simulink library "Power_Electronic_Lab_Controllers"  (R2019b)
settings: Solver=VariableStepAuto  StartTime=0.0  StopTime=10.0  RelTol=1e-3
settings Model: Creator=mehdi  LastModifiedBy=mehdi

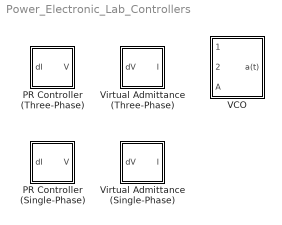
== system Power_Electronic_Lab_Controllers ==
  PR Controller (Single-Phase) : Subsystem  mask{Kp=0.1, Kr=0.2, w0=100*pi}
      mask prompts: Kp "Proportional Gain"; Kr "Resonant Gain"; w0 "Mid Angular Freqeuncy"
      mask DialogControl DescGroupVar Prompt: PR Controller
      mask DialogControl DescTextVar1 Prompt: This Type of controller used as PI Controller but for Sinosoidal input with Angular Freqeunce near by w0.
      mask DialogControl DescTextVar Prompt: The controller desined with 2 parameter Kp and Kr. To understand and desing this controller plot bode diagram from controller transfer function.
  PR Controller (Three-Phase) : Subsystem  mask{Kp=0.1, Kr=0.2, w0=100*pi}
      mask prompts: Kp "Proportional Gain"; Kr "Resonant Gain"; w0 "Mid Angular Freqeuncy"
      mask DialogControl DescGroupVar Prompt: PR Controller
      mask DialogControl DescTextVar1 Prompt: This Type of controller used as PI Controller but for Sinosoidal input with Angular Freqeunce near by w0.
      mask DialogControl DescTextVar Prompt: The controller desined with 2 parameter Kp and Kr. To understand and desing this controller plot bode diagram from controller transfer function.
  VCO : Subsystem  mask{input_sel=Freq. and Arc, pn_sel=Posetive, arc_type_sel=cos, k=-2.0944, theta0=1.5708}
      mask prompts: input_sel "Arc"; pn_sel "Sequence"; arc_type_sel "Function"
      mask TypeOptions input_sel: Arc Only | Freq. Only | Freq. and Arc
      mask Callback input_sel: VCO_Callback()
      mask TypeOptions pn_sel: Posetive | Negetive
      mask Callback pn_sel:
      | sel=get_param(gcb, 'pn_sel');
      | if strcmp(sel, 'Posetive')
      |     set_param(gcb, 'k', num2str(-2*pi/3))
      | else
      |     set_param(gcb, 'k', num2str(+2*pi/3))
      | end
      mask TypeOptions arc_type_sel: sin | cos
      mask Callback arc_type_sel:
      | type=get_param(gcb, 'arc_type_sel');
      | if strcmp(type, 'sin')
      |     set_param(gcb, 'theta0', num2str(0))
      | else
      |     set_param(gcb, 'theta0', num2str(pi/2))
      | end
      mask DialogControl Container2 Prompt: Hidden Parameters
      mask Display:
      | sel=get_param(gcb,  'input_sel');
      | 
      | switch sel
      | case 'Arc Only'
      |     port_label('input', 1, '\theta', 'texmode', 'on')
      | case 'Freq. Only'
      |     port_label('input', 1, '\omega', 'texmode', 'on')
      | case 'Freq. and Arc'
      |     port_label('input', 1, '\theta', 'texmode', 'on')
      |     port_label('input', 2, '\omega', 'texmode', 'on')
      | end
  Virtual Admittance (Single-Phase) : Subsystem  mask{R=0.05, X=0.1, Zb=1.6, w0=100*pi}
      mask prompts: R "R (pu)"; X "X (pu)"; w0 "Angelur Frequency"
      mask DialogControl DescGroupVar Prompt: Virtual Admmitance
      mask DialogControl DescTextVar Prompt: This module is one of control structures of Grig Feeder and used for calculate refrence current from actual voltage of inverter and VCO output.
  Virtual Admittance (Three-Phase) : Subsystem  mask{R=0.05, X=0.1, Zb=1.6, w0=100*pi}
      mask prompts: R "R (pu)"; X "X (pu)"; w0 "Angelur Frequency"
      mask DialogControl DescGroupVar Prompt: Virtual Admmitance
      mask DialogControl DescTextVar Prompt: This module is one of control structures of Grig Feeder and used for calculate refrence current from actual voltage of inverter and VCO output.

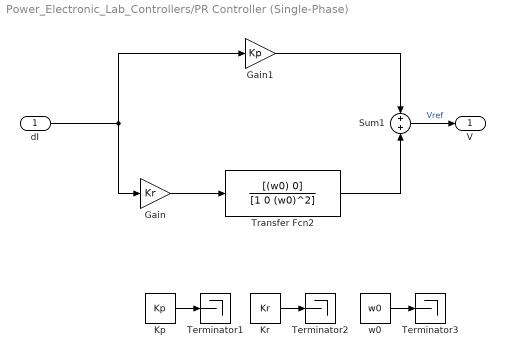
== system Power_Electronic_Lab_Controllers/PR Controller (Single-Phase) ==
  dI : Inport
  Gain : Gain  Gain=Kr
  Gain1 : Gain  Gain=Kp
  Kp : Constant  Value=Kp
  Kr : Constant  Value=Kr
  Sum1 : Sum
  Terminator1 : Terminator
  Terminator2 : Terminator
  Terminator3 : Terminator
  Transfer Fcn2 : TransferFcn  Numerator=[(w0) 0]  Denominator=[1 0 (w0)^2]
  w0 : Constant  Value=w0
  V : Outport  VectorParamsAs1DForOutWhenUnconnected=off
  wires:
  Transfer Fcn2/1 -> Sum1/2
  Gain/1 -> Transfer Fcn2/1
  Kr/1 -> Terminator2/1
  Kp/1 -> Terminator1/1
  w0/1 -> Terminator3/1
  dI/1 -> Gain1/1, Gain/1
  Gain1/1 -> Sum1/1
  Sum1/1 -> V/1  "Vref"

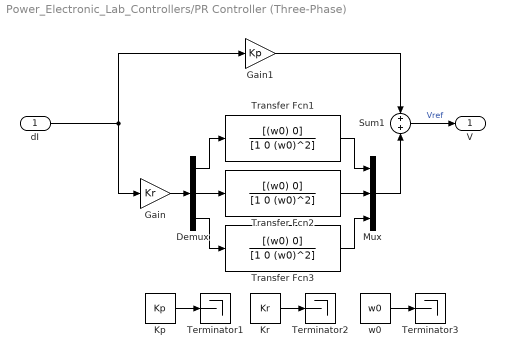
== system Power_Electronic_Lab_Controllers/PR Controller (Three-Phase) ==
  dI : Inport
  Demux : Demux  Outputs=3
  Gain : Gain  Gain=Kr
  Gain1 : Gain  Gain=Kp
  Kp : Constant  Value=Kp
  Kr : Constant  Value=Kr
  Mux : Mux  Inputs=3
  Sum1 : Sum
  Terminator1 : Terminator
  Terminator2 : Terminator
  Terminator3 : Terminator
  Transfer Fcn1 : TransferFcn  Numerator=[(w0) 0]  Denominator=[1 0 (w0)^2]
  Transfer Fcn2 : TransferFcn  Numerator=[(w0) 0]  Denominator=[1 0 (w0)^2]
  Transfer Fcn3 : TransferFcn  Numerator=[(w0) 0]  Denominator=[1 0 (w0)^2]
  w0 : Constant  Value=w0
  V : Outport  VectorParamsAs1DForOutWhenUnconnected=off
  wires:
  Demux/2 -> Transfer Fcn2/1
  Transfer Fcn3/1 -> Mux/3
  Sum1/1 -> V/1  "Vref"
  Demux/3 -> Transfer Fcn3/1
  Gain1/1 -> Sum1/1
  Transfer Fcn2/1 -> Mux/2
  Mux/1 -> Sum1/2
  dI/1 -> Gain/1, Gain1/1
  Gain/1 -> Demux/1
  Transfer Fcn1/1 -> Mux/1
  Demux/1 -> Transfer Fcn1/1
  w0/1 -> Terminator3/1
  Kp/1 -> Terminator1/1
  Kr/1 -> Terminator2/1

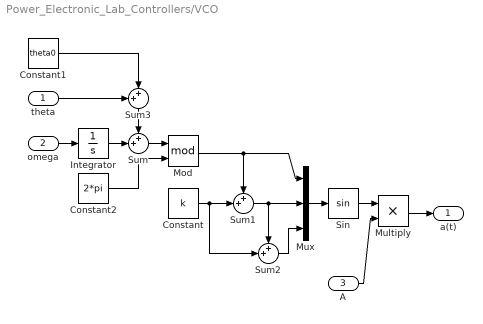
== system Power_Electronic_Lab_Controllers/VCO ==
  theta : Inport
  omega : Inport  Port=2
  A : Inport  Port=3
  Constant : Constant  Value=k
  Constant1 : Constant  Value=theta0
  Constant2 : Constant  Value=2*pi
  Integrator : Integrator
  Mod : Math  Operator=mod  SaturateOnIntegerOverflow=on
  Multiply : Product
  Mux : Mux  Inputs=3
  Sin : Trigonometry
  Sum{,1..3} (4 alike) : Sum  Inputs=++|
  a(t) : Outport  VectorParamsAs1DForOutWhenUnconnected=off
  wires:
  theta/1 -> Sum3/1
  omega/1 -> Integrator/1
  Constant1/1 -> Sum3/2
  Sum3/1 -> Sum/1
  Integrator/1 -> Sum/2
  Sum/1 -> Mod/1
  Mod/1 -> Mux/1, Sum1/1
  Sum2/1 -> Mux/3
  Sin/1 -> Multiply/1
  Mux/1 -> Sin/1
  Sum1/1 -> Sum2/1, Mux/2
  Constant/1 -> Sum1/2, Sum2/2
  Constant2/1 -> Mod/2
  Multiply/1 -> a(t)/1
  A/1 -> Multiply/2

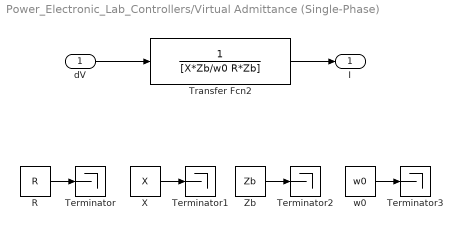
== system Power_Electronic_Lab_Controllers/Virtual Admittance (Single-Phase) ==
  dV : Inport
  R : Constant  Value=R
  Terminator{,1..3} (4 alike) : Terminator
  Transfer Fcn2 : TransferFcn  Numerator=1  Denominator=[X*Zb/w0 R*Zb]
  X : Constant  Value=X
  Zb : Constant  Value=Zb
  w0 : Constant  Value=w0
  I : Outport  VectorParamsAs1DForOutWhenUnconnected=off
  wires:
  Zb/1 -> Terminator2/1
  w0/1 -> Terminator3/1
  X/1 -> Terminator1/1
  R/1 -> Terminator/1
  Transfer Fcn2/1 -> I/1
  dV/1 -> Transfer Fcn2/1

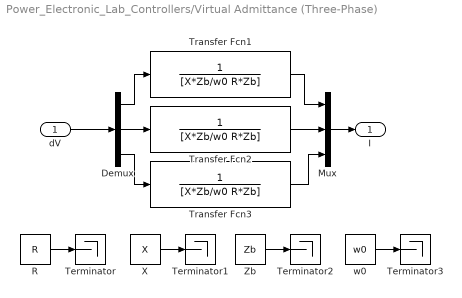
== system Power_Electronic_Lab_Controllers/Virtual Admittance (Three-Phase) ==
  dV : Inport
  Demux : Demux  Outputs=3
  Mux : Mux  Inputs=3
  R : Constant  Value=R
  Terminator{,1..3} (4 alike) : Terminator
  Transfer Fcn1 : TransferFcn  Numerator=1  Denominator=[X*Zb/w0 R*Zb]
  Transfer Fcn2 : TransferFcn  Numerator=1  Denominator=[X*Zb/w0 R*Zb]
  Transfer Fcn3 : TransferFcn  Numerator=1  Denominator=[X*Zb/w0 R*Zb]
  X : Constant  Value=X
  Zb : Constant  Value=Zb
  w0 : Constant  Value=w0
  I : Outport  VectorParamsAs1DForOutWhenUnconnected=off
  wires:
  Demux/1 -> Transfer Fcn1/1
  Transfer Fcn1/1 -> Mux/1
  Mux/1 -> I/1
  dV/1 -> Demux/1
  R/1 -> Terminator/1
  X/1 -> Terminator1/1
  w0/1 -> Terminator3/1
  Zb/1 -> Terminator2/1
  Transfer Fcn2/1 -> Mux/2
  Transfer Fcn3/1 -> Mux/3
  Demux/3 -> Transfer Fcn3/1
  Demux/2 -> Transfer Fcn2/1
